simulink model "lyuEinspurmodell_ISIS_2016A"  (R2016a)
settings: Solver=ode1  StartTime=0.0  StopTime=SIM_time  FixedStep=1e-3  RelTol=1e-3
values from neighbouring files (symbols this model uses):
  Bf = 10.96    [lyutemplate_steuerung.m]
  Br = 12.67    [lyutemplate_steuerung.m]
  cf = 60000    [lyutemplate_steuerung.m]
  Cf = 1.1    [lyutemplate_steuerung.m]
  cr = 75000    [lyutemplate_steuerung.m]
  Cr = 1.3    [lyutemplate_steuerung.m]
  Fzeta0 = 8000    [lyutemplate_steuerung.m]
  Fzetaf = fzg_m*g*lh/l    (= 11216.8604651)    [lyutemplate_steuerung.m]
  Fzetar = fzg_m*g*(l-lh)/l    (= 6146.83953488)    [lyutemplate_steuerung.m]
  fzg_Jz = 1752    [lyutemplate_steuerung.m]
  fzg_m = 1770    [lyutemplate_steuerung.m]
  iL = 14    [lyutemplate_steuerung.m]
  k_Fzeta = 0.25    [lyutemplate_steuerung.m]
  lh = 1.75    [lyutemplate_steuerung.m]
  lv = (l-lh)    (= 0.959)    [lyutemplate_steuerung.m]
  manoever_choice = 1    [lyutemplate_steuerung.m]
  mu = 1.05    [lyutemplate_steuerung.m]
  speed = 10    [lyutemplate_steuerung.m]
  steering_angle = 30*pi/180    (= 0.523598775598)    [lyutemplate_steuerung.m]
  tire_choice = 0    [lyutemplate_steuerung.m]
undefined symbols (not defined in the file or in its folder): sinus_freq
settings Model: Creator=TWeiskircher  LastModifiedBy=Jason
settings DataIOCC: LimitDataPoints=on  SaveFormat=Array  SignalLoggingSaveFormat=ModelDataLogs
settings OptimizationCC: ExpressionDepthLimit=2147483647
settings DebuggingCC: UnderspecifiedInitializationDetection=Classic  MergeDetectMultiDrivingBlocksExec=none  SolverPrmCheckMsg=warning  FcnCallInpInsideContextMsg=EnableAllAsWarning  StateNameClashWarn=warning
settings HardwareCC: ProdBitPerPointer=32  ProdLargestAtomicFloat=None  ProdIntDivRoundTo=Undefined  ProdEndianess=Unspecified  ProdWordSize=32  ProdHWDeviceType=32-bit Generic
settings ModelReferenceCC: PropagateSignalLabelsOutOfModel=off
settings GRTTargetCC: CombineOutputUpdateFcns=off  GRTInterface=on

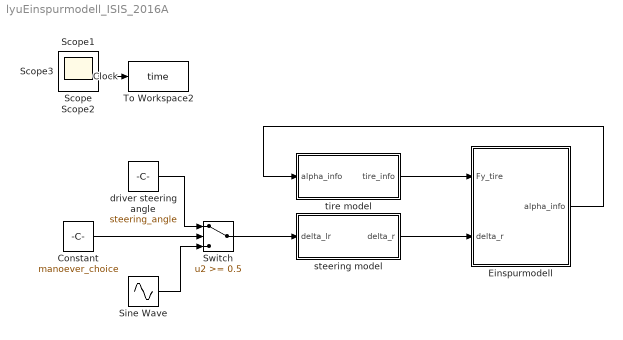
== system lyuEinspurmodell_ISIS_2016A ==
  Clock : Clock
  Constant : Constant  Value=manoever_choice
  Einspurmodell : Subsystem
  Sine Wave : Sin  Amplitude=steering_angle  Frequency=sinus_freq*2*pi  SampleTime=0
  Switch : Switch  Threshold=0.5
  To Workspace2 : ToWorkspace  VariableName=time  SampleTime=-1
  driver steering angle : Constant  Value=steering_angle
  steering model : Subsystem
  tire model : Subsystem
  Scope{,1..3} (4 alike) : Scope
  wires:
  steering model/1(delta_r) -> Einspurmodell/2(delta_r)
  tire model/1(tire_info) -> Einspurmodell/1(Fy_tire)
  Einspurmodell/1(alpha_info) -> tire model/1(alpha_info)
  Clock/1 -> To Workspace2/1
  Switch/1 -> steering model/1(delta_lr)
  Constant/1 -> Switch/2
  driver steering angle/1 -> Switch/1
  Sine Wave/1 -> Switch/3

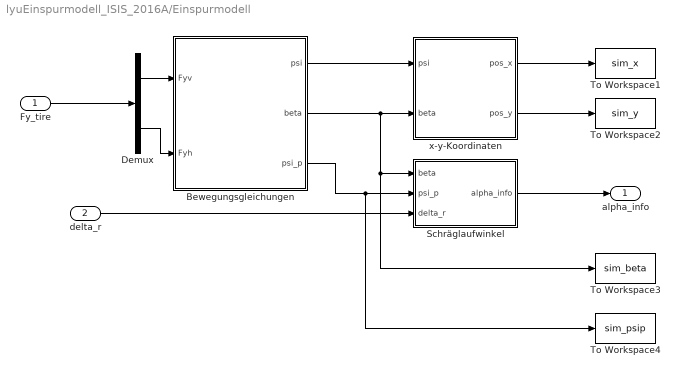
== system lyuEinspurmodell_ISIS_2016A/Einspurmodell ==
  Fy_tire : Inport
  delta_r : Inport  Port=2
  Bewegungsgleichungen : Subsystem
  Demux : Demux  Outputs=2
  Schräglaufwinkel : Subsystem
  To Workspace1 : ToWorkspace  VariableName=sim_x  SampleTime=-1
  To Workspace2 : ToWorkspace  VariableName=sim_y  SampleTime=-1
  To Workspace3 : ToWorkspace  VariableName=sim_beta  SampleTime=-1
  To Workspace4 : ToWorkspace  VariableName=sim_psip  SampleTime=-1
  x-y-Koordinaten : Subsystem
  alpha_info : Outport
  wires:
  Fy_tire/1 -> Demux/1
  Demux/1 -> Bewegungsgleichungen/1(Fyv)
  Demux/2 -> Bewegungsgleichungen/2(Fyh)
  delta_r/1 -> Schräglaufwinkel/3(delta_r)
  Bewegungsgleichungen/1(psi) -> x-y-Koordinaten/1(psi)
  Bewegungsgleichungen/2(beta) -> x-y-Koordinaten/2(beta), Schräglaufwinkel/1(beta), To Workspace3/1
  Schräglaufwinkel/1(alpha_info) -> alpha_info/1
  Bewegungsgleichungen/3(psi_p) -> Schräglaufwinkel/2(psi_p), To Workspace4/1
  x-y-Koordinaten/1(pos_x) -> To Workspace1/1
  x-y-Koordinaten/2(pos_y) -> To Workspace2/1

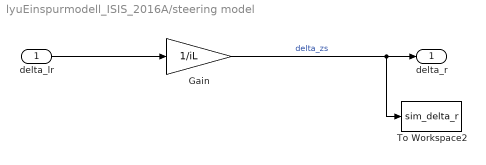
== system lyuEinspurmodell_ISIS_2016A/steering model ==
  delta_lr : Inport
  Gain : Gain  Gain=1/iL
  To Workspace2 : ToWorkspace  VariableName=sim_delta_r  SampleTime=-1
  delta_r : Outport
  wires:
  delta_lr/1 -> Gain/1
  Gain/1 -> To Workspace2/1, delta_r/1  "delta_zs"

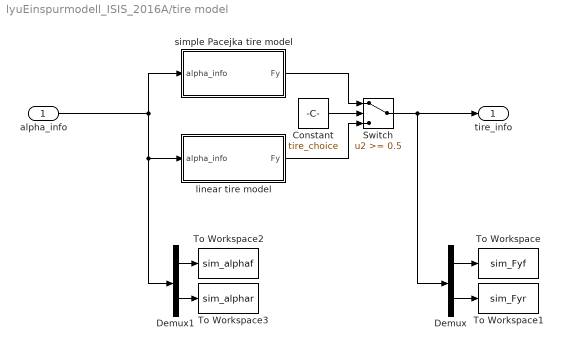
== system lyuEinspurmodell_ISIS_2016A/tire model ==
  alpha_info : Inport
  Constant : Constant  Value=tire_choice
  Demux : Demux  Outputs=2
  Demux1 : Demux  Outputs=2
  Switch : Switch  Threshold=0.5
  To Workspace : ToWorkspace  VariableName=sim_Fyf  SampleTime=-1
  To Workspace1 : ToWorkspace  VariableName=sim_Fyr  SampleTime=-1
  To Workspace2 : ToWorkspace  VariableName=sim_alphaf  SampleTime=-1
  To Workspace3 : ToWorkspace  VariableName=sim_alphar  SampleTime=-1
  linear tire model : MATLAB Function  TreatAsAtomicUnit=on
  simple Pacejka tire model : MATLAB Function  TreatAsAtomicUnit=on
  tire_info : Outport
  wires:
  alpha_info/1 -> simple Pacejka tire model/1(alpha_info), Demux1/1, linear tire model/1(alpha_info)
  Constant/1 -> Switch/2
  simple Pacejka tire model/1(Fy) -> Switch/1
  linear tire model/1(Fy) -> Switch/3
  Switch/1 -> tire_info/1, Demux/1
  Demux/1 -> To Workspace/1
  Demux/2 -> To Workspace1/1
  Demux1/1 -> To Workspace2/1
  Demux1/2 -> To Workspace3/1

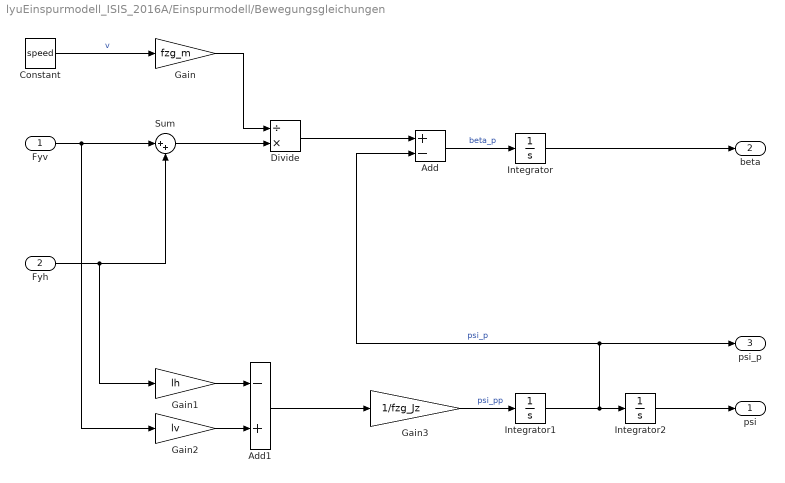
== system lyuEinspurmodell_ISIS_2016A/Einspurmodell/Bewegungsgleichungen ==
  Fyv : Inport
  Fyh : Inport  Port=2
  Add : Sum  Inputs=+-
  Add1 : Sum  Inputs=-+
  Constant : Constant  Value=speed
  Divide : Product  Inputs=/*
  Gain : Gain  Gain=fzg_m
  Gain1 : Gain  Gain=lh
  Gain2 : Gain  Gain=lv
  Gain3 : Gain  Gain=1/fzg_Jz
  Integrator : Integrator
  Integrator1 : Integrator
  Integrator2 : Integrator
  Sum : Sum  Inputs=|++
  psi : Outport
  beta : Outport  Port=2
  psi_p : Outport  Port=3
  wires:
  Fyh/1 -> Gain1/1, Sum/2
  Fyv/1 -> Gain2/1, Sum/1
  Sum/1 -> Divide/2
  Constant/1 -> Gain/1  "v"
  Gain/1 -> Divide/1
  Divide/1 -> Add/1
  Integrator1/1 -> psi_p/1, Add/2, Integrator2/1  "psi_p"
  Add/1 -> Integrator/1  "beta_p"
  Integrator/1 -> beta/1
  Gain1/1 -> Add1/1
  Gain2/1 -> Add1/2
  Add1/1 -> Gain3/1
  Gain3/1 -> Integrator1/1  "psi_pp"
  Integrator2/1 -> psi/1

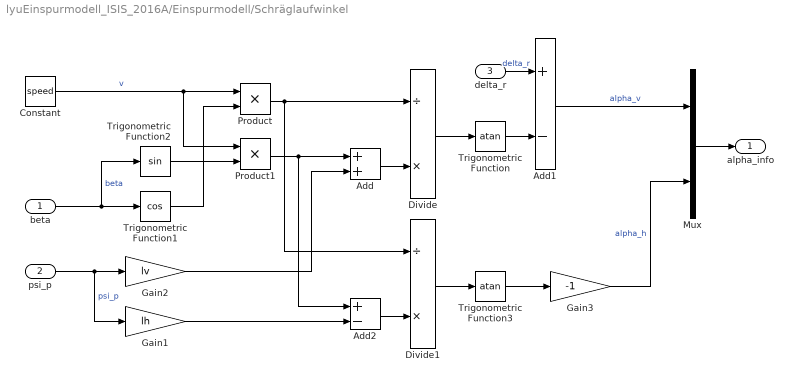
== system lyuEinspurmodell_ISIS_2016A/Einspurmodell/Schräglaufwinkel ==
  beta : Inport
  psi_p : Inport  Port=2
  delta_r : Inport  Port=3
  Add : Sum
  Add1 : Sum  Inputs=+-
  Add2 : Sum  Inputs=+-
  Constant : Constant  Value=speed
  Divide : Product  Inputs=/*
  Divide1 : Product  Inputs=/*
  Gain1 : Gain  Gain=lh
  Gain2 : Gain  Gain=lv
  Gain3 : Gain  Gain=-1
  Mux : Mux  Inputs=2
  Product : Product
  Product1 : Product
  Trigonometric Function : Trigonometry  Operator=atan
  Trigonometric Function1 : Trigonometry  Operator=cos
  Trigonometric Function2 : Trigonometry
  Trigonometric Function3 : Trigonometry  Operator=atan
  alpha_info : Outport
  wires:
  Mux/1 -> alpha_info/1
  beta/1 -> Trigonometric Function2/1, Trigonometric Function1/1  "beta"
  Constant/1 -> Product1/1, Product/1  "v"
  Trigonometric Function1/1 -> Product/2
  Trigonometric Function2/1 -> Product1/2
  psi_p/1 -> Gain1/1, Gain2/1  "psi_p"
  Product1/1 -> Add2/1, Add/1
  Gain2/1 -> Add/2
  Add/1 -> Divide/2
  Product/1 -> Divide1/1, Divide/1
  Divide/1 -> Trigonometric Function/1
  Trigonometric Function/1 -> Add1/2
  delta_r/1 -> Add1/1  "delta_r"
  Add1/1 -> Mux/1  "alpha_v"
  Divide1/1 -> Trigonometric Function3/1
  Gain1/1 -> Add2/2
  Add2/1 -> Divide1/2
  Trigonometric Function3/1 -> Gain3/1
  Gain3/1 -> Mux/2  "alpha_h"

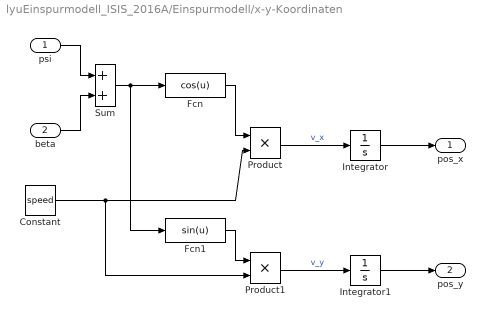
== system lyuEinspurmodell_ISIS_2016A/Einspurmodell/x-y-Koordinaten ==
  psi : Inport
  beta : Inport  Port=2
  Constant : Constant  Value=speed
  Fcn : Fcn  Expr=cos(u)
  Fcn1 : Fcn  Expr=sin(u)
  Integrator : Integrator
  Integrator1 : Integrator
  Product : Product  RndMeth=Zero
  Product1 : Product  RndMeth=Zero
  Sum : Sum
  pos_x : Outport
  pos_y : Outport  Port=2
  wires:
  Constant/1 -> Product/2, Product1/2
  Fcn/1 -> Product/1
  Product/1 -> Integrator/1  "v_x"
  psi/1 -> Sum/1
  beta/1 -> Sum/2
  Sum/1 -> Fcn/1, Fcn1/1
  Fcn1/1 -> Product1/1
  Product1/1 -> Integrator1/1  "v_y"
  Integrator/1 -> pos_x/1
  Integrator1/1 -> pos_y/1

== matlab function lyuEinspurmodell_ISIS_2016A/tire model/linear tire model ==
  data: alpha_info input size=2; Fy output size=2; mu parameter; cf parameter; cr parameter; Fzetaf parameter; Fzetar parameter
function Fy = fcn(alpha_info, mu, cf, cr, Fzetaf, Fzetar)
%#eml

slipf = alpha_info(1);
slipr = alpha_info(2);

% Calculate Fmax:
Fmaxf = mu*Fzetaf;
Fmaxr = mu*Fzetar;

% Calculate slip curves
Fyf = mu * cf * slipf;
Fyr = mu * cr * slipr;

% % test on frition circle limit:(unzulässig, da sonst Probleme bei Schwimmwinkelberechnung)
% if abs(Fyf) > Fmaxf
%     Fyf = sign(Fyf)*Fmaxf;
% end
% 
% if abs(Fyr) > Fmaxr
%     Fyr = sign(Fyr)*Fmaxr;
% end

Fy = [Fyf; Fyr];

== matlab function lyuEinspurmodell_ISIS_2016A/tire model/simple Pacejka tire model ==
  data: alpha_info input size=2; Fy output size=2; mu parameter; Cf parameter; Cr parameter; Bf parameter; Br parameter; Fzetaf parameter; Fzetar parameter; Fzeta0 parameter; k_Fzeta parameter
function Fy = fcn(alpha_info, mu, Cf, Cr, Bf, Br, Fzetaf, Fzetar, Fzeta0, k_Fzeta)
%#eml

dummy = [0; 0];


Fy = dummy;
